simulink model "series"  (R2024b)
settings: Solver=VariableStepAuto  StartTime=0.0  StopTime=100  RelTol=1e-3
undefined symbols (not defined in the file or in its folder): a, magnitude
libraries: dspindex x1, dspsrcs4 x1
settings Model: Creator=keshm  LastModifiedBy=keshm

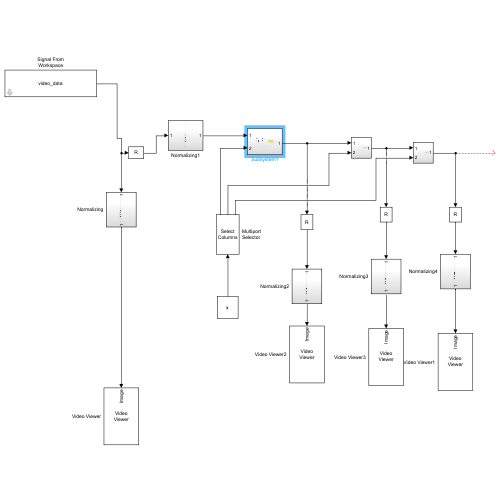
[thumbnail: Simulink's stored preview of the top-level diagram]
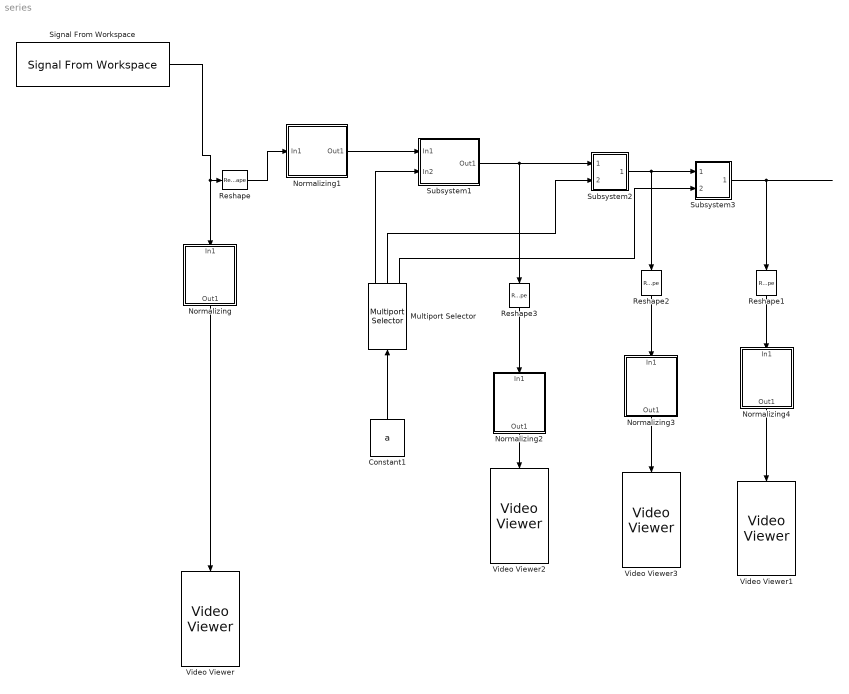
== system series ==
  Constant1 : Constant  Value=a
  Multiport Selector : dspindex/Multiport Selector  rowsOrCols=Columns  idxCellArray={1,2,3}  idxErrMode=Clip Index
      settings: LibrarySourceBlock=|
      | dsphdlsupportsigmgmt/Multiport
      | Selector
  Normalizing : Subsystem
  Normalizing1 : Subsystem
  Normalizing2 : Subsystem
  Normalizing3 : Subsystem
  Normalizing4 : Subsystem
  Reshape : Reshape  OutputDimensionality=Customize  OutputDimensions=[524288,1]
  Reshape1 : Reshape  OutputDimensionality=Customize  OutputDimensions=[1024,512]
  Reshape2 : Reshape  OutputDimensionality=Customize  OutputDimensions=[1024,512]
  Reshape3 : Reshape  OutputDimensionality=Customize  OutputDimensions=[1024,512]
  Signal From Workspace : dspsrcs4/Signal From Workspace  X=video_data  Ts=1  nsamps=1  OutputAfterFinalValue=Setting to zero  ignoreOrWarnInputAndFrameLengths=off  OutputFrames=off
  Subsystem1 : Subsystem
  Subsystem2 : Subsystem
  Subsystem3 : Subsystem
  Video Viewer : VideoViewer  FigPos=[769.8 813.2 766.4 300]
  Video Viewer1 : VideoViewer  FigPos=[1.8 813.2 766.4 708]
  Video Viewer2 : VideoViewer  FigPos=[1.8 813.2 766.4 708]
  Video Viewer3 : VideoViewer  FigPos=[-63.8 823.6 766.4 708]
  wires:
  Signal From Workspace/1 -> Normalizing/1(In1), Reshape/1
  Constant1/1 -> Multiport Selector/1
  Reshape/1 -> Normalizing1/1(In1)
  Multiport Selector/1 -> Subsystem1/2(In2)
  Subsystem3/1(Out1) -> Reshape1/1
  Subsystem1/1(Out1) -> Subsystem2/1(In1), Reshape3/1
  Reshape3/1 -> Normalizing2/1(In1)
  Subsystem2/1(Out1) -> Subsystem3/1(In1), Reshape2/1
  Reshape2/1 -> Normalizing3/1(In1)
  Normalizing/1(Out1) -> Video Viewer/1
  Normalizing1/1(Out1) -> Subsystem1/1(In1)
  Reshape1/1 -> Normalizing4/1(In1)
  Normalizing2/1(Out1) -> Video Viewer2/1
  Normalizing3/1(Out1) -> Video Viewer3/1
  Normalizing4/1(Out1) -> Video Viewer1/1
  Multiport Selector/2 -> Subsystem2/2(In2)
  Multiport Selector/3 -> Subsystem3/2(In2)

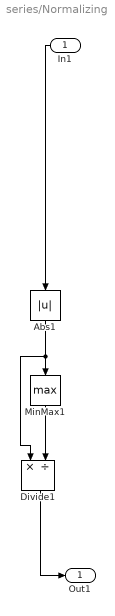
== system series/Normalizing ==
  In1 : Inport
  Abs1 : Abs  SaturateOnIntegerOverflow=off
  Divide1 : Product  Inputs=*/
  MinMax1 : MinMax  Function=max
  Out1 : Outport
  wires:
  Abs1/1 -> Divide1/1, MinMax1/1
  In1/1 -> Abs1/1
  MinMax1/1 -> Divide1/2
  Divide1/1 -> Out1/1

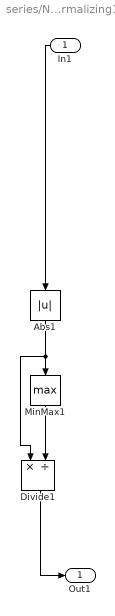
== system series/Normalizing1 ==
  In1 : Inport
  Abs1 : Abs  SaturateOnIntegerOverflow=off
  Divide1 : Product  Inputs=*/
  MinMax1 : MinMax  Function=max
  Out1 : Outport
  wires:
  Abs1/1 -> Divide1/1, MinMax1/1
  In1/1 -> Abs1/1
  MinMax1/1 -> Divide1/2
  Divide1/1 -> Out1/1

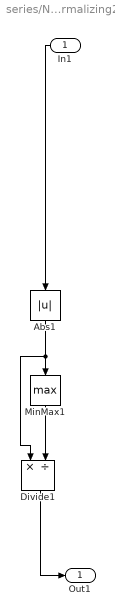
== system series/Normalizing2 ==
  In1 : Inport
  Abs1 : Abs  SaturateOnIntegerOverflow=off
  Divide1 : Product  Inputs=*/
  MinMax1 : MinMax  Function=max
  Out1 : Outport
  wires:
  Abs1/1 -> Divide1/1, MinMax1/1
  In1/1 -> Abs1/1
  MinMax1/1 -> Divide1/2
  Divide1/1 -> Out1/1

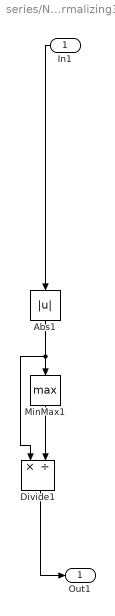
== system series/Normalizing3 ==
  In1 : Inport
  Abs1 : Abs  SaturateOnIntegerOverflow=off
  Divide1 : Product  Inputs=*/
  MinMax1 : MinMax  Function=max
  Out1 : Outport
  wires:
  Abs1/1 -> Divide1/1, MinMax1/1
  In1/1 -> Abs1/1
  MinMax1/1 -> Divide1/2
  Divide1/1 -> Out1/1

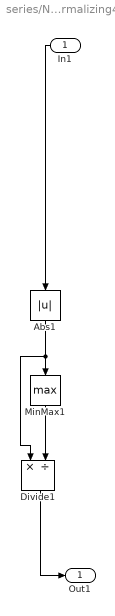
== system series/Normalizing4 ==
  In1 : Inport
  Abs1 : Abs  SaturateOnIntegerOverflow=off
  Divide1 : Product  Inputs=*/
  MinMax1 : MinMax  Function=max
  Out1 : Outport
  wires:
  Abs1/1 -> Divide1/1, MinMax1/1
  In1/1 -> Abs1/1
  MinMax1/1 -> Divide1/2
  Divide1/1 -> Out1/1

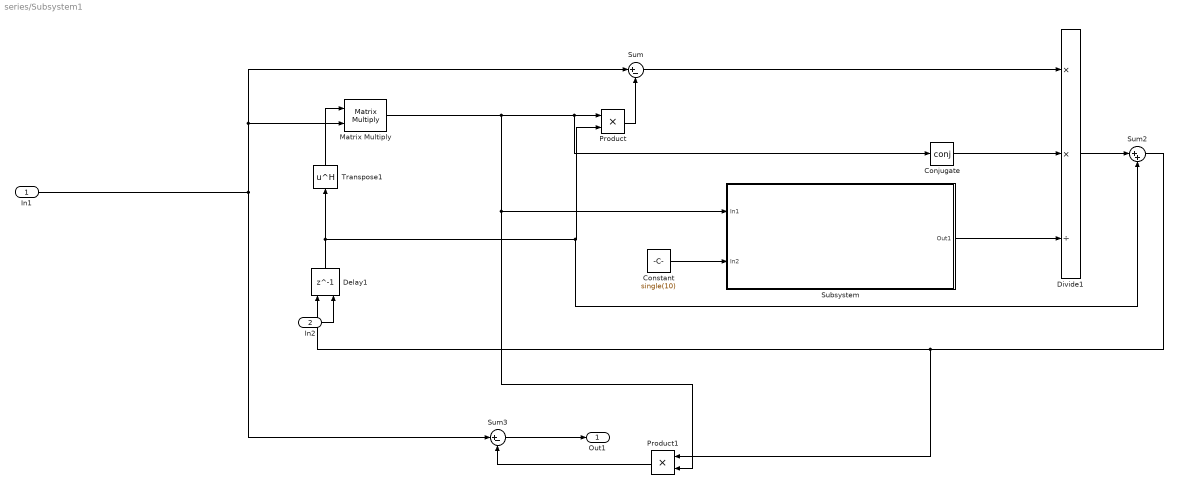
== system series/Subsystem1 ==
  In1 : Inport
  In2 : Inport  Port=2
  Conjugate : Math  Operator=conj  SignedPower=on  RndMeth=Zero
  Constant : Constant  Value=single(10)
  Delay1 : Delay  DelayLength=1  InitialConditionSource=Input port  InitialCondition=0
      settings: InputPortMap=u0,p4
  Divide1 : Product  Inputs=**/
  Matrix Multiply : Product  Multiplication=Matrix(*)
  Product : Product
  Product1 : Product
  Subsystem : Subsystem
  Sum : Sum  Inputs=|+-
  Sum2 : Sum  Inputs=|++
  Sum3 : Sum  Inputs=|+-
  Transpose1 : Math  Operator=hermitian
  Out1 : Outport
  wires:
  In1/1 -> Sum3/1, Matrix Multiply/2, Sum/1
  Subsystem/1(Out1) -> Divide1/3
  Delay1/1 -> Transpose1/1, Product/2, Sum2/2
  Matrix Multiply/1 -> Product/1, Conjugate/1, Product1/2, Subsystem/1(In1)
  Sum2/1 -> Delay1/1, Product1/1
  Constant/1 -> Subsystem/2(In2)
  Divide1/1 -> Sum2/1
  Transpose1/1 -> Matrix Multiply/1
  Sum/1 -> Divide1/1
  Product/1 -> Sum/2
  Conjugate/1 -> Divide1/2
  Product1/1 -> Sum3/2
  In2/1 -> Delay1/2
  Sum3/1 -> Out1/1

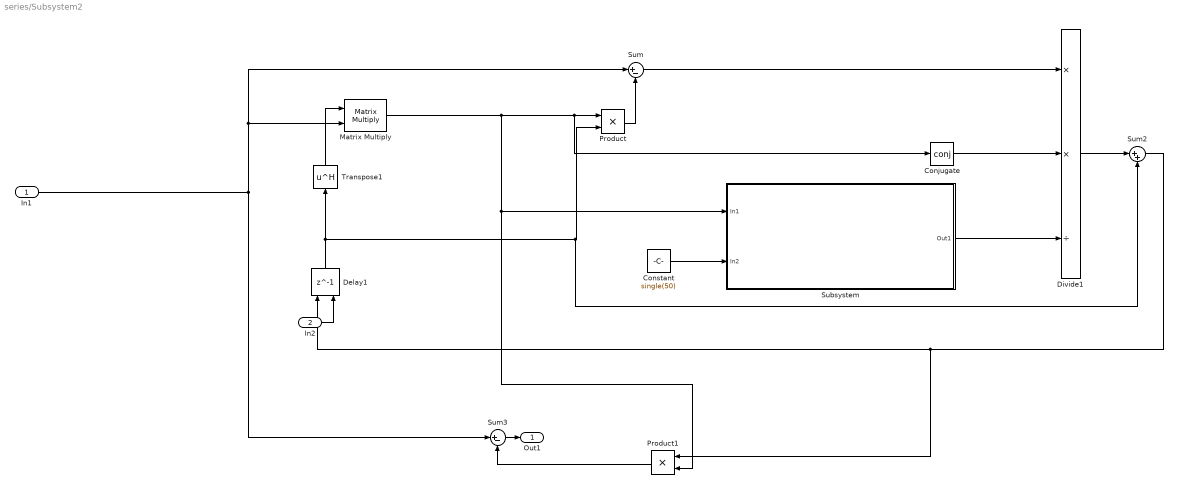
== system series/Subsystem2 ==
  In1 : Inport
  In2 : Inport  Port=2
  Conjugate : Math  Operator=conj  SignedPower=on  RndMeth=Zero
  Constant : Constant  Value=single(50)
  Delay1 : Delay  DelayLength=1  InitialConditionSource=Input port  InitialCondition=0
      settings: InputPortMap=u0,p4
  Divide1 : Product  Inputs=**/
  Matrix Multiply : Product  Multiplication=Matrix(*)
  Product : Product
  Product1 : Product
  Subsystem : Subsystem
  Sum : Sum  Inputs=|+-
  Sum2 : Sum  Inputs=|++
  Sum3 : Sum  Inputs=|+-
  Transpose1 : Math  Operator=hermitian
  Out1 : Outport
  wires:
  In1/1 -> Sum3/1, Matrix Multiply/2, Sum/1
  Subsystem/1(Out1) -> Divide1/3
  Delay1/1 -> Transpose1/1, Product/2, Sum2/2
  Matrix Multiply/1 -> Product/1, Conjugate/1, Product1/2, Subsystem/1(In1)
  Sum2/1 -> Delay1/1, Product1/1
  Constant/1 -> Subsystem/2(In2)
  Divide1/1 -> Sum2/1
  Transpose1/1 -> Matrix Multiply/1
  Sum/1 -> Divide1/1
  Product/1 -> Sum/2
  Conjugate/1 -> Divide1/2
  Product1/1 -> Sum3/2
  In2/1 -> Delay1/2
  Sum3/1 -> Out1/1

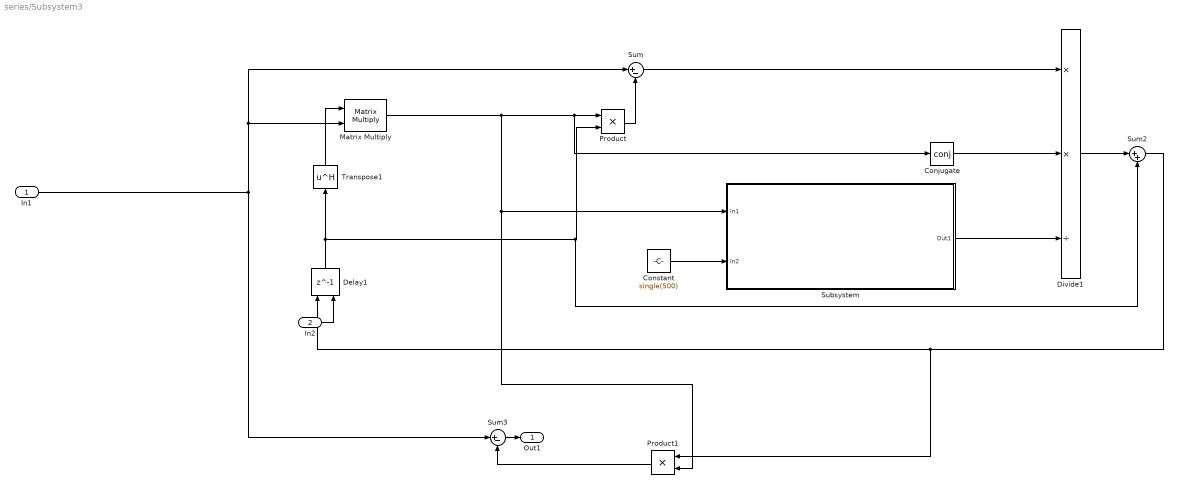
== system series/Subsystem3 ==
  In1 : Inport
  In2 : Inport  Port=2
  Conjugate : Math  Operator=conj  SignedPower=on  RndMeth=Zero
  Constant : Constant  Value=single(500)
  Delay1 : Delay  DelayLength=1  InitialConditionSource=Input port  InitialCondition=0
      settings: InputPortMap=u0,p4
  Divide1 : Product  Inputs=**/
  Matrix Multiply : Product  Multiplication=Matrix(*)
  Product : Product
  Product1 : Product
  Subsystem : Subsystem
  Sum : Sum  Inputs=|+-
  Sum2 : Sum  Inputs=|++
  Sum3 : Sum  Inputs=|+-
  Transpose1 : Math  Operator=hermitian
  Out1 : Outport
  wires:
  In1/1 -> Sum3/1, Matrix Multiply/2, Sum/1
  Subsystem/1(Out1) -> Divide1/3
  Delay1/1 -> Transpose1/1, Product/2, Sum2/2
  Matrix Multiply/1 -> Product/1, Conjugate/1, Product1/2, Subsystem/1(In1)
  Sum2/1 -> Delay1/1, Product1/1
  Constant/1 -> Subsystem/2(In2)
  Divide1/1 -> Sum2/1
  Transpose1/1 -> Matrix Multiply/1
  Sum/1 -> Divide1/1
  Product/1 -> Sum/2
  Conjugate/1 -> Divide1/2
  Product1/1 -> Sum3/2
  In2/1 -> Delay1/2
  Sum3/1 -> Out1/1

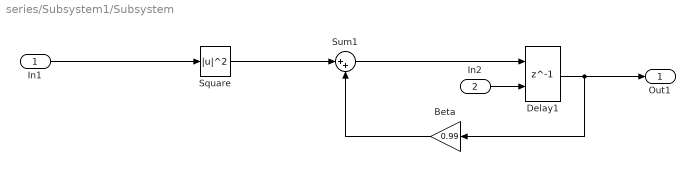
== system series/Subsystem1/Subsystem ==
  In1 : Inport
  In2 : Inport  Port=2
  Beta : Gain  Gain=0.99
  Delay1 : Delay  DelayLength=1  InitialConditionSource=Input port  InitialCondition=0
      settings: InputPortMap=u0,p4
  Square : Math  Operator=magnitude^2
  Sum1 : Sum  Inputs=|++
  Out1 : Outport
  wires:
  Square/1 -> Sum1/1
  Beta/1 -> Sum1/2
  In1/1 -> Square/1
  Delay1/1 -> Beta/1, Out1/1
  In2/1 -> Delay1/2
  Sum1/1 -> Delay1/1

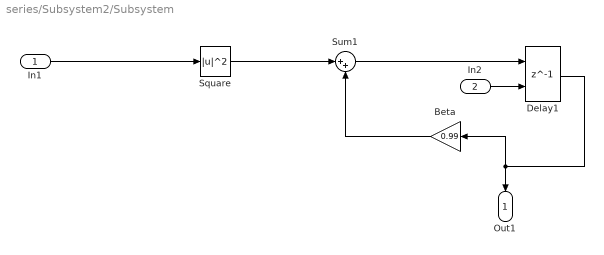
== system series/Subsystem2/Subsystem ==
  In1 : Inport
  In2 : Inport  Port=2
  Beta : Gain  Gain=0.99
  Delay1 : Delay  DelayLength=1  InitialConditionSource=Input port  InitialCondition=0
      settings: InputPortMap=u0,p4
  Square : Math  Operator=magnitude^2
  Sum1 : Sum  Inputs=|++
  Out1 : Outport
  wires:
  Square/1 -> Sum1/1
  Beta/1 -> Sum1/2
  In1/1 -> Square/1
  Delay1/1 -> Beta/1, Out1/1
  In2/1 -> Delay1/2
  Sum1/1 -> Delay1/1

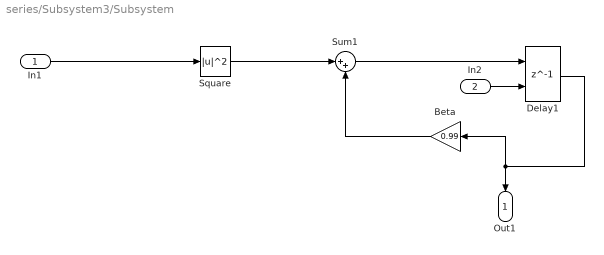
== system series/Subsystem3/Subsystem ==
  In1 : Inport
  In2 : Inport  Port=2
  Beta : Gain  Gain=0.99
  Delay1 : Delay  DelayLength=1  InitialConditionSource=Input port  InitialCondition=0
      settings: InputPortMap=u0,p4
  Square : Math  Operator=magnitude^2
  Sum1 : Sum  Inputs=|++
  Out1 : Outport
  wires:
  Square/1 -> Sum1/1
  Beta/1 -> Sum1/2
  In1/1 -> Square/1
  Delay1/1 -> Beta/1, Out1/1
  In2/1 -> Delay1/2
  Sum1/1 -> Delay1/1
